simulink model "experiment203"  (R2018b)
settings: Solver=VariableStepAuto  StartTime=0.0  StopTime=10.0  RelTol=1e-3
settings Model: Creator=HIT-QJ  LastModifiedBy=HIT-QJ

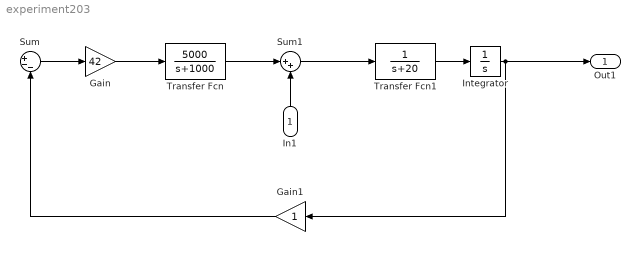
== system experiment203 ==
  In1 : Inport
  Gain : Gain  Gain=42
  Gain1 : Gain
  Integrator : Integrator
  Sum : Sum  Inputs=|+--
  Sum1 : Sum  Inputs=|++
  Transfer Fcn : TransferFcn  Numerator=[5000]  Denominator=[1 1000]
  Transfer Fcn1 : TransferFcn  Denominator=[1 20]
  Out1 : Outport
  wires:
  In1/1 -> Sum1/2
  Transfer Fcn/1 -> Sum1/1
  Sum1/1 -> Transfer Fcn1/1
  Transfer Fcn1/1 -> Integrator/1
  Integrator/1 -> Gain1/1, Out1/1
  Gain1/1 -> Sum/3
  Sum/1 -> Gain/1
  Gain/1 -> Transfer Fcn/1
